simulink model "NonlinearModel1"  (R2021b)
settings: Solver=ode23t  StartTime=0.0  StopTime=200  RelTol=1e-3
values from neighbouring files (symbols this model uses):
  A3 = [1  0  0; 0  1  0; 0  0  1]    [Final model.mat]
  D = eye(3).*k_e    [Init.m]    (also in Test.m)
  I_s = 1.464*10^-5    (= 1.464e-05)    [Init.m]
  Ib = diag([0.0021; 0.0023;0.0024])    [Init.m]
  Initq_bob = [1,0,0,0]    [Init.m]    (also in Test.m = [1 0 0 0])
  J = Ib - A3*I_s*A3.'    [Init.m]
  k_e = 0.3    [Init.m]    (also in Test.m)
  startup = false    [Init.m]    (also in Test.m)
  startup1 = false    [Init.m]
  w_0 = sqrt(mu/rc^3)    [Init.m]
  Wbob = [1.4; 1; 1.5]    [Init.m]
  wsinit = zeros(3,1)    [Init.m]
libraries: simulink_extras x4, sharedtransform x1
settings Model: Creator=Lenovo  LastModifiedBy=Lenovo

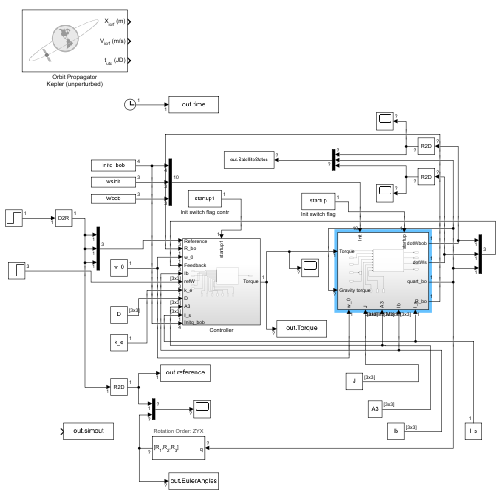
[thumbnail: Simulink's stored preview of the top-level diagram]
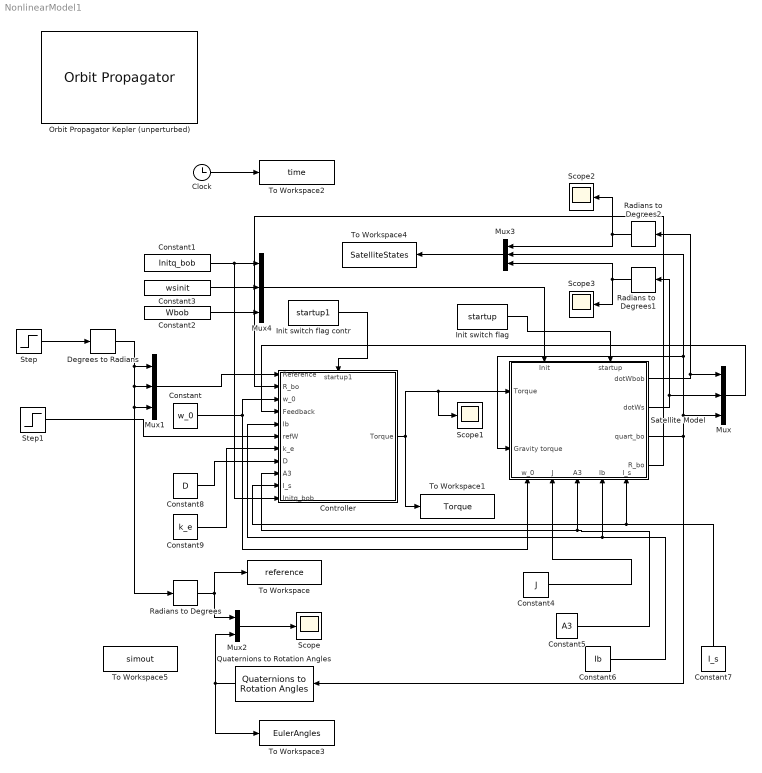
== system NonlinearModel1 ==
  Clock : Clock
  Constant : Constant  Value=w_0
  Constant1 : Constant  Value=Initq_bob
  Constant2 : Constant  Value=Wbob
  Constant3 : Constant  Value=wsinit
  Constant4 : Constant  Value=J
  Constant5 : Constant  Value=A3
  Constant6 : Constant  Value=Ib
  Constant7 : Constant  Value=I_s
  Constant8 : Constant  Value=D
  Constant9 : Constant  Value=k_e
  Controller : Subsystem
      settings: PortSchema="{\"entries\":[{\"content\":{\"sides\":[{\"content\":{\"connectorIds\":[\"In1\",\"In2\",\"In3\",\"In4\",\"In5\",\"In6\",\"In7\",\"In8\",\"In9\",\"In10\",\"In11\"]},\"type\":\"ConnectorPlacement.EquallySpacedRectSide\",\"uuid\":\"5590ad9e-04f9-4af7-9b4f-f6478cf6a2ce\"},{\"content\":{\"connectorIds\":[\"Out1\"],\"side\":\"RIGHT\"},\"type\":\"ConnectorPlacement.EquallySpacedRectSide\",\"uuid\":\"ce5d6df3-1bbd-4344-9f78-59de01b16bbe\"},{\"content\":{\"connectorIds\":[\"In12\"],\"side\":\"TOP\"},\"type\":\"ConnectorPlacement.EquallySpacedRectSide\",\"uuid\":\"46d2e6ad-14c9-4352-aed1-d0491a069da7\"}]},\"type\":\"ConnectorPlacement.EquallySpacedConnector\",\"uuid\":\"3cf07d37-360f-4057-a8fd-56cec6ac6e5f\"}],\"packageUris\":[\"http://schema.mathworks.com/mf0/Connector/R2020b\"],\"version\":\"1.0\"}"
  Degrees to Radians : simulink_extras/Transformations/Degrees to Radians
  Init switch flag : Constant  Value=startup
  Init switch flag contr : Constant  Value=startup1
  Mux{,1,3..4} (4 alike) : Mux  Inputs=3
  Mux2 : Mux  Inputs=2
  Orbit Propagator Kepler (unperturbed) : OrbitPropagator  inertialPosition=[3649700.0 3308200.0 -4676600.0]  inertialVelocity=[-2750.8 6666.4 2573.4]  fixedPosition=[-4142689.0 -2676864.7 -4669861.6]  fixedVelocity=[1452.7 -6720.7 2568.1]  customR=3396200  customMu=4.305e13  customJ2=1.0826269e-03  customOmega=4.06125949e-3
  Quaternions to Rotation Angles : sharedtransform/Quaternions to Rotation Angles  rotationOrder=ZYX  aMode=aMode
      settings: SourceProductBaseCode=AE,PW,DR,MT,UV,VE
  Radians to Degrees : simulink_extras/Transformations/Radians to Degrees
  Radians to Degrees1 : simulink_extras/Transformations/Radians to Degrees
  Radians to Degrees2 : simulink_extras/Transformations/Radians to Degrees
  Satellite Model : Subsystem
      settings: PortSchema="{\"entries\":[{\"content\":{\"sides\":[{\"content\":{\"connectorIds\":[\"In1\",\"In2\"]},\"type\":\"ConnectorPlacement.EquallySpacedRectSide\",\"uuid\":\"ed600d3a-bd99-4e9e-b304-9a2a6bbc0ab4\"},{\"content\":{\"connectorIds\":[\"Out1\",\"Out2\",\"Out3\",\"Out4\"],\"side\":\"RIGHT\"},\"type\":\"ConnectorPlacement.EquallySpacedRectSide\",\"uuid\":\"702358d8-c789-483d-bed3-4e4bb7a14f25\"},{\"content\":{\"connectorIds\":[\"In3\",\"In4\"],\"side\":\"TOP\"},\"type\":\"ConnectorPlacement.EquallySpacedRectSide\",\"uuid\":\"76bd57d9-d6cb-4206-8221-b8f97d7bca63\"},{\"content\":{\"connectorIds\":[\"In5\",\"In6\",\"In7\",\"In8\",\"In9\"],\"side\":\"BOTTOM\"},\"type\":\"ConnectorPlacement.EquallySpacedRectSide\",\"uuid\":\"b2771b37-9ece-425f-9236-ba4802dbc464\"}]},\"type\":\"ConnectorPlacement.EquallySpacedConnector\",\"uuid\":\"6eb2613a-d71e-4315-b1b1-4843921ec110\"}],\"packageUris\":[\"http://schema.mathworks.com/mf0/Connector/R2020b\"],\"version\":\"1.0\"}"
  Scope{,1..3} (4 alike) : Scope
  Step : Step  Time=0  After=60  SampleTime=0
  Step1 : Step  After=[1; 2; 3]  SampleTime=0
  To Workspace : ToWorkspace  VariableName=reference  SampleTime=-1
  To Workspace1 : ToWorkspace  VariableName=Torque  SampleTime=-1
  To Workspace2 : ToWorkspace  VariableName=time  SampleTime=-1
  To Workspace3 : ToWorkspace  VariableName=EulerAngles  SampleTime=-1
  To Workspace4 : ToWorkspace  VariableName=SatelliteStates  SaveFormat=Timeseries  SampleTime=-1
  To Workspace5 : ToWorkspace  VariableName=simout  SaveFormat=Timeseries  SampleTime=-1
  wires:
  Step/1 -> Degrees to Radians/1
  Degrees to Radians/1 -> Mux1/1, Mux1/3, Radians to Degrees/1, Mux1/2
  Mux1/1 -> Controller/1(Reference)
  Controller/1(Torque) -> Scope1/1, Satellite Model/1(Torque), To Workspace1/1
  Satellite Model/1(dotWbob) -> Mux/1, Radians to Degrees2/1
  Satellite Model/2(dotWs) -> Mux/2, Radians to Degrees1/1
  Satellite Model/3(quart_bo) -> Satellite Model/2(Gravity torque), Mux3/2, Mux/3, Quaternions to Rotation Angles/1
  Mux/1 -> Controller/4(Feedback)
  Satellite Model/4(R_bo) -> Controller/2(R_bo)
  Mux2/1 -> Scope/1
  Radians to Degrees/1 -> To Workspace/1, Mux2/1
  Quaternions to Rotation Angles/1 -> Mux2/2, To Workspace3/1
  Clock/1 -> To Workspace2/1
  Radians to Degrees1/1 -> Scope3/1, Mux3/3
  Radians to Degrees2/1 -> Mux3/1, Scope2/1
  Mux3/1 -> To Workspace4/1
  Constant/1 -> Satellite Model/5(w_0), Controller/3(w_0)
  Constant1/1 -> Controller/11(Initq_bob), Mux4/1
  Constant3/1 -> Mux4/2
  Constant2/1 -> Mux4/3
  Mux4/1 -> Satellite Model/3(Init)
  Init switch flag/1 -> Satellite Model/4(startup)
  Constant4/1 -> Satellite Model/6(J)
  Constant5/1 -> Controller/9(A3), Satellite Model/7(A3)
  Constant6/1 -> Controller/5(Ib), Satellite Model/8(Ib)
  Constant7/1 -> Controller/10(I_s), Satellite Model/9(I_s)
  Constant8/1 -> Controller/8(D)
  Constant9/1 -> Controller/7(k_e)
  Step1/1 -> Controller/6(refW)
  Init switch flag contr/1 -> Controller/12(startup1)

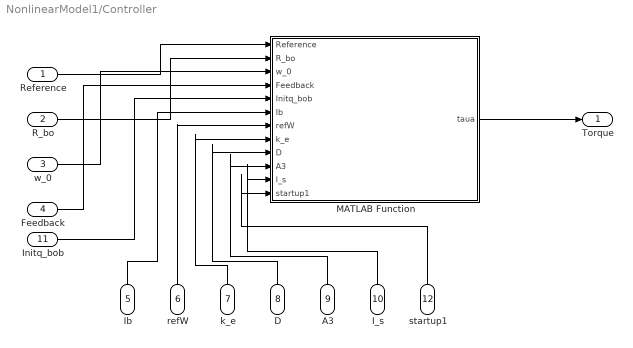
== system NonlinearModel1/Controller ==
  Reference : Inport
  R_bo : Inport  Port=2
  w_0 : Inport  Port=3
  Feedback : Inport  Port=4
  Ib : Inport  Port=5
  refW : Inport  Port=6
  k_e : Inport  Port=7
  D : Inport  Port=8
  A3 : Inport  Port=9
  I_s : Inport  Port=10
  Initq_bob : Inport  Port=11
  startup1 : Inport  Port=12
  MATLAB Function : MATLAB Function  TreatAsAtomicUnit=on
  Torque : Outport
  wires:
  R_bo/1 -> MATLAB Function/2(R_bo)
  MATLAB Function/1(taua) -> Torque/1
  Reference/1 -> MATLAB Function/1(Reference)
  w_0/1 -> MATLAB Function/3(w_0)
  Feedback/1 -> MATLAB Function/4(Feedback)
  Ib/1 -> MATLAB Function/6(Ib)
  refW/1 -> MATLAB Function/7(refW)
  k_e/1 -> MATLAB Function/8(k_e)
  D/1 -> MATLAB Function/9(D)
  A3/1 -> MATLAB Function/10(A3)
  I_s/1 -> MATLAB Function/11(I_s)
  Initq_bob/1 -> MATLAB Function/5(Initq_bob)
  startup1/1 -> MATLAB Function/12(startup1)

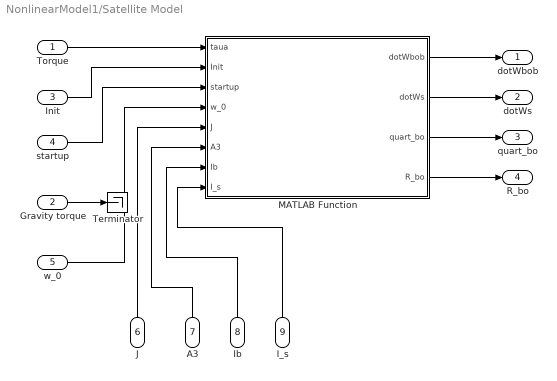
== system NonlinearModel1/Satellite Model ==
  Torque : Inport
  Gravity torque : Inport  Port=2
  Init : Inport  Port=3
  startup : Inport  Port=4
  w_0 : Inport  Port=5
  J : Inport  Port=6
  A3 : Inport  Port=7
  Ib : Inport  Port=8
  I_s : Inport  Port=9
  MATLAB Function : MATLAB Function  TreatAsAtomicUnit=on
  Terminator : Terminator
  dotWbob : Outport
  dotWs : Outport  Port=2
  quart_bo : Outport  Port=3
  R_bo : Outport  Port=4
  wires:
  Torque/1 -> MATLAB Function/1(taua)
  Gravity torque/1 -> Terminator/1
  MATLAB Function/1(dotWbob) -> dotWbob/1
  MATLAB Function/2(dotWs) -> dotWs/1
  MATLAB Function/3(quart_bo) -> quart_bo/1
  MATLAB Function/4(R_bo) -> R_bo/1
  Init/1 -> MATLAB Function/2(Init)
  startup/1 -> MATLAB Function/3(startup)
  w_0/1 -> MATLAB Function/4(w_0)
  A3/1 -> MATLAB Function/6(A3)
  J/1 -> MATLAB Function/5(J)
  Ib/1 -> MATLAB Function/7(Ib)
  I_s/1 -> MATLAB Function/8(I_s)

== matlab function NonlinearModel1/Satellite Model/MATLAB Function ==
  data: taua input; dotWbob output; dotWs output; quart_bo output; R_bo output; Init input; startup input; w_0 input; J input; A3 input; Ib input; I_s input
function [dotWbob,dotWs,quart_bo,R_bo] = SystemNonlinearModel(taua,Init,startup,w_0,J,A3,Ib,I_s)
% Function that calculates the system states
%   This system function receives initializing input parameters and control
%   signals and calculates the components of the ordinal differential
%   equations of each state.

quaternions = zeros(1,4);
AngVel = zeros(3,1);
WAngVel = zeros(3,1);
Initq_bob = Init(1:4);
n = Initq_bob(1);
e1 = Initq_bob(2);
e2 = Initq_bob(3);
e3 = Initq_bob(4);
% Decide whether to use initial values or the one calculated in the
% previous itteration
if(startup == true)
    Initq_bob = Init(1:4);
    n = Initq_bob(1);
    e1 = Initq_bob(2);
    e2 = Initq_bob(3);
    e3 = Initq_bob(4);

    R_bo = [1-2*e2^2-2*e3^2 2*e1*e2-2*e3*n 2*e1*e3+2*e2*n;
        2*e1*e2+2*e3*n 1-2*e1^2-2*e3^2 2*e2*e3-2*e1*n;
        2*e1*e3-2*e2*n 2*e2*e3+2*e1*n 1-2*e1^2-2*e2^2];
    c_2 = R_bo(:,2);
    c_3 = R_bo(:,3);

    Ws = Init(5:7);
    ws1 = Ws(1);
    ws2 = Ws(2);
    ws3 = Ws(3);
    wbob = Init(8:10);


else
    q_bob = quaternions;
    n = q_bob(1);
    e1 = q_bob(2);
    e2 = q_bob(3);
    e3 = q_bob(4);

    R_bo = [1-2*e2^2-2*e3^2 2*e1*e2-2*e3*n 2*e1*e3+2*e2*n;
        2*e1*e2+2*e3*n 1-2*e1^2-2*e3^2 2*e2*e3-2*e1*n;
        2*e1*e3-2*e2*n 2*e2*e3+2*e1*n 1-2*e1^2-2*e2^2];
    c_2 = R_bo(:,2);
    c_3 = R_bo(:,3);

    ws1 = WAngVel(1);
    ws2 = WAngVel(2);
    ws3 = WAngVel(3);
    wbob = AngVel;
end
%EndInit

M1 = eye(3);
wbib = wbob - w_0*c_2;

% The angular velocity of the satellite ode

fhi = J\(-cross(wbib,(Ib*wbib+A3(:,1)*I_s.*ws1+A3(:,2)*I_s.*ws2+A3(:,3)*I_s.*ws3)));%inertial component equation
fht = -J\A3*taua;                     %input torque equation
fhg = J\(3*w_0^2*cross(c_3,Ib*c_3));     %gravitational component equation
dotc = -cross(wbob,c_2);
fha = dotc*(w_0);                      %additional (orbital velocity component)

dotWbob = fhi+fht+fhg+dotc+fha;
% The reaction wheel angular velocity ode

fsi = A3'*(J\(cross(wbib,(Ib*wbib+A3(:,1)*I_s.*ws1+A3(:,2)*I_s.*ws2+A3(:,3)*I_s.*ws3))));%mod to accomodate ws
fst = (A3'*(J\A3)+1/I_s)*taua;
fsg = -A3'*(J\(3*w_0^2*cross(c_3,Ib*c_3)));

dotWs = fsi+fst+fsg;
ws1 = dotWs(1);
ws2 = dotWs(2);
ws3 = dotWs(3);

% update quaternion positioning
e = [e1; e2; e3]
dot_n = -1/2*e'*dotWbob;
dot_e = 1/2*(n*M1*dotWbob + cross(e,dotWbob));

quart_bo = [dot_n; dot_e];
e1 = dot_e(1);
e2 = dot_e(2);
e3 = dot_e(3);

% update rotation matrix

R_bo = [1-2*e2^2-2*e3^2 2*e1*e2-2*e3*dot_n 2*e1*e3+2*e2*dot_n;
    2*e1*e2+2*e3*dot_n 1-2*e1^2-2*e3^2 2*e2*e3-2*e1*dot_n;
    2*e1*e3-2*e2*dot_n 2*e2*e3+2*e1*dot_n 1-2*e1^2-2*e2^2];

% update calculated data

quaternions = quart_bo;
AngVel = dotWbob;
WAngVel = dotWs;

%update flag
startup = false;

end

== matlab function NonlinearModel1/Controller/MATLAB Function ==
  data: Reference input; taua output; R_bo input; w_0 input; Feedback input; Initq_bob input; Ib input; refW input; k_e input; D input; A3 input; I_s input; startup1 input
function taua = LyapunovController1(Reference, R_bo, w_0, Feedback, Initq_bob, Ib, refW, k_e, D, A3, I_s, startup1)

%Lyapunov controller function 
%   Control strategy based on a Lyapunov function candidate. The core idea
%   is that the reaction wheel angular velocity is interpreted as an
%   external control input and is therefore not included in the statespace
%   of the system.
if(startup1 == false)
    dotWbob = [0 0 0];
    dotWs = [0 0 0];
    quart_bo = [1 0 0 0];
    u = zeros(3,1);
else   
    dotWbob = Feedback(1:3)';
    dotWs = Feedback(4:7)';
    quart_bo = Feedback(8:10);
end
M = ones(3,1);
% Angular error rate
refWdot = -Ib^-1*cross(refW,(Ib*refW))+Ib^-1*u;
deltaW = dotWbob-refW;
deltaWdot = -Ib^-1*deltaW.*cross(refW,Ib*M)-cross(deltaW,(Ib*refW))-Ib^-1*cross(deltaW,(Ib*deltaW))+Ib^-1*u-refWdot-Ib^-1*cross(refW,(Ib*dotWbob));
%
% Quaternion error

qref = eul2quat(Reference');
refinv = quatinv(qref);
deltaq = quatmultiply(quart_bo',refinv);
deltaq_4 = deltaq(1);                   %deltaq_4 is in fact the first element but is named for math model analogy
deltaq_v = deltaq(2:4);

deltaq_vdot = (1/2).*(-cross(deltaW,deltaq_v)-2.*cross(deltaW,deltaq_v)+deltaq_4*deltaW);
deltaq_4dot = -(1/2).*deltaW.'.*deltaq_v;
deltaq_dot = [deltaq_4dot,deltaq_vdot];

%



dot_n = deltaq_dot(1);
e1 = deltaq_dot(2);
e2 = deltaq_dot(3);
e3 = deltaq_dot(4);

% calculate error (REFERENCE-FEEDBACK)

% Look into quaternion error

% Update DCM with the calculated error parameters
R_bo = [1-2*e2^2-2*e3^2 2*e1*e2-2*e3*dot_n 2*e1*e3+2*e2*dot_n;
         2*e1*e2+2*e3*dot_n 1-2*e1^2-2*e3^2 2*e2*e3-2*e1*dot_n;
         2*e1*e3-2*e2*dot_n 2*e2*e3+2*e1*dot_n 1-2*e1^2-2*e2^2];

c_2 = R_bo(:,2);
c_3 = R_bo(:,3);

taua = k_e.*deltaq_vdot' + D*deltaWdot + w_0.*cross(c_2,A3*I_s*(A3'*deltaWdot+dotWs)) - w_0^2*cross(c_2,Ib*c_2)+3*w_0^2*cross(c_3,Ib*c_3);
u = taua;
end
